simulink model "blender"  (Simulink 8.7)
settings: Solver=ode45  StartTime=0.0  StopTime=10.0  RelTol=1e-3
undefined symbols (not defined in the file or in its folder): blendTime
libraries: WBCLibrary x2
settings Model: Creator=luca  LastModifiedBy=gnava
settings DebuggingCC: UnderspecifiedInitializationDetection=Simplified  MergeDetectMultiDrivingBlocksExec=error  SolverPrmCheckMsg=warning
settings ConfigComp: CovSFcnEnable=off

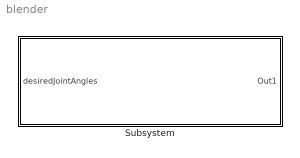
== system blender ==
  Subsystem : Subsystem

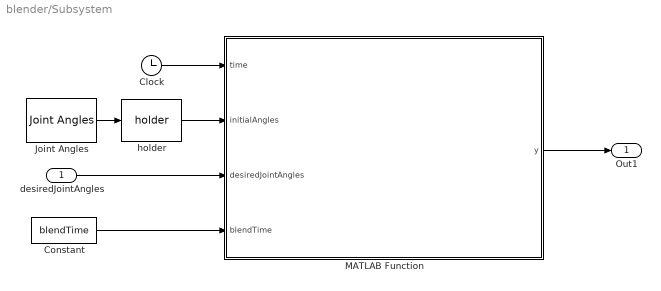
== system blender/Subsystem ==
  desiredJointAngles : Inport
  Clock : Clock
  Constant : Constant  Value=blendTime
  Joint Angles : WBCLibrary/wholeBodyStates/Joint Angles  robotName=robotName  localName=localName
  MATLAB Function : MATLAB Function  TreatAsAtomicUnit=on
  "holder " : WBCLibrary/Utilities/holder 
  Out1 : Outport
  wires:
  Constant/1 -> MATLAB Function/4(blendTime)
  Joint Angles/1 -> "holder "/1
  desiredJointAngles/1 -> MATLAB Function/3(desiredJointAngles)
  MATLAB Function/1(y) -> Out1/1
  Clock/1 -> MATLAB Function/1(time)
  "holder "/1 -> MATLAB Function/2(initialAngles)

== matlab function Subsystem/MATLAB Function ==
  data: time input double; y output double; initialAngles input double; desiredJointAngles input double; blendTime input double
function y = fcn(time, initialAngles, desiredJointAngles, blendTime)

if time < blendTime
    y = initialAngles + (desiredJointAngles - initialAngles) * (time / blendTime); 
else
    y = desiredJointAngles;
end
